simulink model "trailer_kinetic"  (R2018a)
settings: Solver=ode45  StartTime=0.0  StopTime=sim_time  RelTol=1e-3
values from neighbouring files (symbols this model uses):
  A = M \ K    [kinetic_trailer.m]
  a2 = 6.2941    [kinetic_trailer.m]
  B = M \ N    [kinetic_trailer.m]
  C = eye(6)    [kinetic_trailer.m]
  D = zeros(6, 1)    [kinetic_trailer.m]
  h1 = 2.9691    [kinetic_trailer.m]
  ICs = [0; deg2rad(0); deg2rad(0); deg2rad(0); y_IC; deg2rad(270)]    [kinetic_trailer.m]
  K = (-1 / v) * [(C1+C2+C3)              (C1*a1 - C2*b1 - C3*(h1+L2) + (m1+m2)*v.^2)          (-C3*L2)     (-C3*v)   0       0 ... (first row only)    [kinetic_trailer.m]
  L1 = a1 + b1    (= 5.7336)    [kinetic_trailer.m]
  tractorIC = [trailerIC(1), trailerIC(2) - (a2+h1)]    [kinetic_trailer.m]
  v = 25    [kinetic_trailer.m]
undefined symbols (not defined in the file or in its folder): L
settings Model: Creator=journ  LastModifiedBy=journeyman

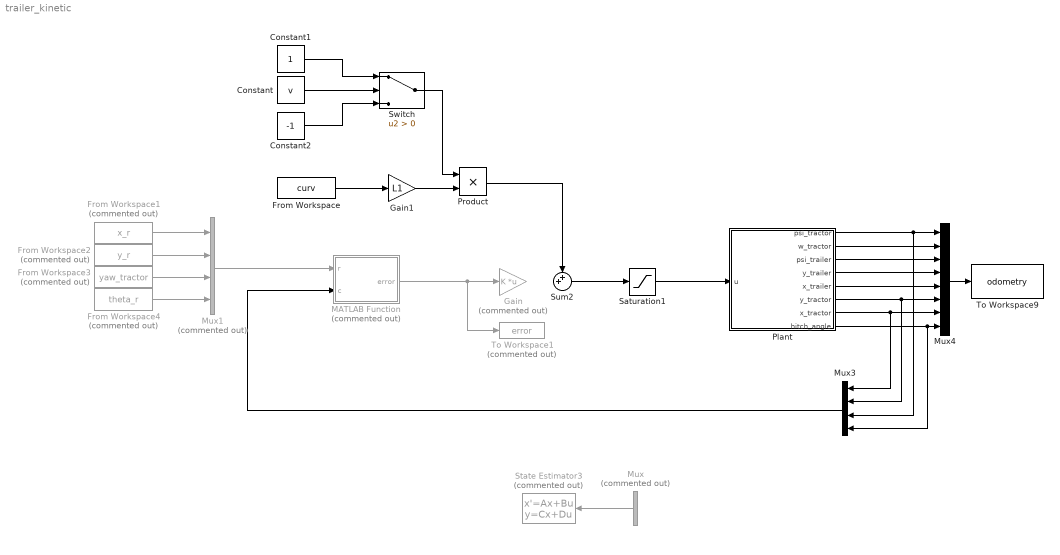
== system trailer_kinetic ==
  Constant : Constant  Value=v
  Constant1 : Constant
  Constant2 : Constant  Value=-1
  From Workspace : FromWorkspace  VariableName=curv  SampleTime=0
  From Workspace1 : FromWorkspace  Commented=on  VariableName=x_r  SampleTime=0  OutputAfterFinalValue=Holding final value
  From Workspace2 : FromWorkspace  Commented=on  VariableName=y_r  SampleTime=0
  From Workspace3 : FromWorkspace  Commented=on  VariableName=yaw_tractor  SampleTime=0
  From Workspace4 : FromWorkspace  Commented=on  VariableName=theta_r  SampleTime=0
  Gain : Gain  Commented=on  Gain=K  Multiplication=Matrix(K*u)
  Gain1 : Gain  Gain=L1
  MATLAB Function : MATLAB Function  Commented=on  TreatAsAtomicUnit=on
  Mux : Mux  Commented=on  Inputs=2
  Mux1 : Mux  Commented=on
  Mux3 : Mux
  Mux4 : Mux  Inputs=8
  Plant : Subsystem
  Product : Product
  Saturation1 : Saturate  UpperLimit=deg2rad(30)  LowerLimit=-deg2rad(30)
  State Estimator3 : StateSpace  Commented=on  A=A - L*C  B=[B L]  C=eye(4)  D=zeros(4,3)  InitialCondition=ICs
  Sum2 : Sum  Inputs=++|
  Switch : Switch  Criteria=u2 > Threshold
  To Workspace1 : ToWorkspace  Commented=on  VariableName=error  SampleTime=-1
  To Workspace9 : ToWorkspace  VariableName=odometry  SampleTime=-1
  wires:
  From Workspace3/1 -> Mux1/3
  Constant1/1 -> Switch/1
  Switch/1 -> Product/1
  From Workspace4/1 -> Mux1/4
  Constant2/1 -> Switch/3
  From Workspace/1 -> Gain1/1
  Sum2/1 -> Saturation1/1
  From Workspace1/1 -> Mux1/1
  From Workspace2/1 -> Mux1/2
  Mux/1 -> State Estimator3/1
  Gain1/1 -> Product/2
  Mux1/1 -> MATLAB Function/1(r)
  MATLAB Function/1(error) -> To Workspace1/1, Gain/1
  Mux3/1 -> MATLAB Function/2(c)
  Constant/1 -> Switch/2
  Mux4/1 -> To Workspace9/1
  Saturation1/1 -> Plant/1(u)
  Plant/1(psi_tractor) -> Mux3/3, Mux4/1
  Plant/2(w_tractor) -> Mux4/2
  Plant/3(psi_trailer) -> Mux4/3
  Plant/4(y_trailer) -> Mux4/4
  Plant/5(x_trailer) -> Mux4/5
  Plant/6(y_tractor) -> Mux3/2, Mux4/6
  Plant/7(x_tractor) -> Mux3/1, Mux4/7
  Plant/8(hitch_angle) -> Mux3/4, Mux4/8
  Product/1 -> Sum2/1

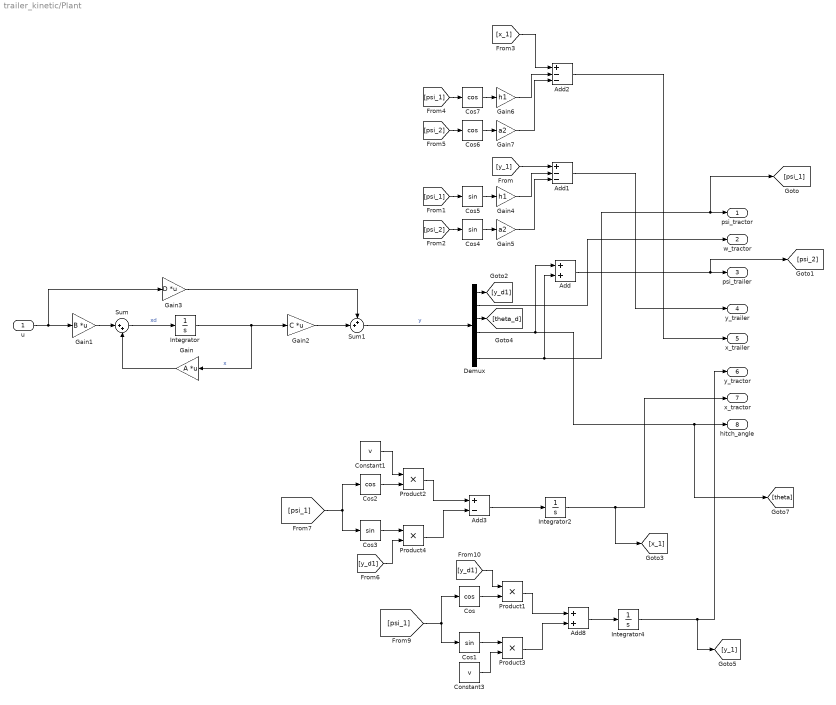
== system trailer_kinetic/Plant ==
  u : Inport
  Add : Sum
  Add1 : Sum  Inputs=+--
  Add2 : Sum  Inputs=+--
  Add3 : Sum  Inputs=+-
  Add8 : Sum
  Constant1 : Constant  Value=v
  Constant3 : Constant  Value=v
  Cos{,2,6..7} (4 alike) : Trigonometry  Operator=cos
  Cos{1,3..5} (4 alike) : Trigonometry
  Demux : Demux  Outputs=6
  Gain : Gain  Gain=A  Multiplication=Matrix(K*u)
  Gain1 : Gain  Gain=B  Multiplication=Matrix(K*u)
  Gain2 : Gain  Gain=C  Multiplication=Matrix(K*u)
  Gain3 : Gain  Gain=D  Multiplication=Matrix(K*u)
  Gain4 : Gain  Gain=h1
  Gain5 : Gain  Gain=a2
  Gain6 : Gain  Gain=h1
  Gain7 : Gain  Gain=a2
  Integrator : Integrator  InitialCondition=ICs
  Integrator2 : Integrator  InitialCondition=tractorIC(1)
  Integrator4 : Integrator  InitialCondition=tractorIC(2)
  Product{1..4} (4 alike) : Product
  Sum : Sum  Inputs=|++
  Sum1 : Sum  Inputs=++|
  psi_tractor : Outport
  w_tractor : Outport  Port=2
  psi_trailer : Outport  Port=3
  y_trailer : Outport  Port=4
  x_trailer : Outport  Port=5
  y_tractor : Outport  Port=6
  x_tractor : Outport  Port=7
  hitch_angle : Outport  Port=8
  wires:
  Integrator/1 -> Gain/1, Gain2/1  "x"
  Gain/1 -> Sum/2
  Gain1/1 -> Sum/1
  Sum/1 -> Integrator/1  "xd"
  Sum1/1 -> Demux/1  "y"
  Gain3/1 -> Sum1/1
  u/1 -> Gain3/1, Gain1/1
  Gain2/1 -> Sum1/2
  Demux/2 -> w_tractor/1
  Demux/4 -> Add/1, [theta], hitch_angle/1
  Add/1 -> [psi_2], psi_trailer/1
  Demux/6 -> Add/2, [psi_1], psi_tractor/1
  Demux/1 -> [y_d1]
  Add3/1 -> Integrator2/1
  Add8/1 -> Integrator4/1
  Integrator4/1 -> [y_1], y_tractor/1
  Demux/3 -> [theta_d]
  [psi_1] -> Cos1/1, Cos/1
  Cos/1 -> Product1/2
  [y_d1] -> Product1/1
  Constant3/1 -> Product3/2
  Cos1/1 -> Product3/1
  Product3/1 -> Add8/2
  Product1/1 -> Add8/1
  Product2/1 -> Add3/1
  Product4/1 -> Add3/2
  Cos3/1 -> Product4/1
  Cos2/1 -> Product2/2
  [psi_1] -> Cos2/1, Cos3/1
  Constant1/1 -> Product2/1
  [y_d1] -> Product4/2
  Add1/1 -> y_trailer/1
  [y_1] -> Add1/1
  Gain4/1 -> Add1/2
  Gain5/1 -> Add1/3
  Integrator2/1 -> [x_1], x_tractor/1
  Add2/1 -> x_trailer/1
  Cos4/1 -> Gain5/1
  [psi_2] -> Cos4/1
  [psi_1] -> Cos5/1
  Cos5/1 -> Gain4/1
  [x_1] -> Add2/1
  Cos7/1 -> Gain6/1
  [psi_1] -> Cos7/1
  [psi_2] -> Cos6/1
  Cos6/1 -> Gain7/1
  Gain7/1 -> Add2/3
  Gain6/1 -> Add2/2

== matlab function trailer_kinetic/MATLAB Function ==
  data: r input; error output; c input
function error = safeminus(r, c)
    error = zeros(3, 1);
    error(1, 1) = r(4) - c(4);
    error(2, 1) = r(2) - c(2);
    
    cross = cos(c(3))*sin(r(3)) - sin(c(3))*cos(r(3));
    dot = cos(c(3))*cos(r(3)) + sin(c(3))*sin(r(3));
    error(3, 1) = atan2(cross, dot);
    
    % error = [theta_e, d1_e, psi1_e]
